simulink model "iBLF"  (R2015b)
settings: Solver=VariableStepAuto  StartTime=0.0  StopTime=10.0  RelTol=1e-3
settings Model: Creator=raghavv  LastModifiedBy=raghavv

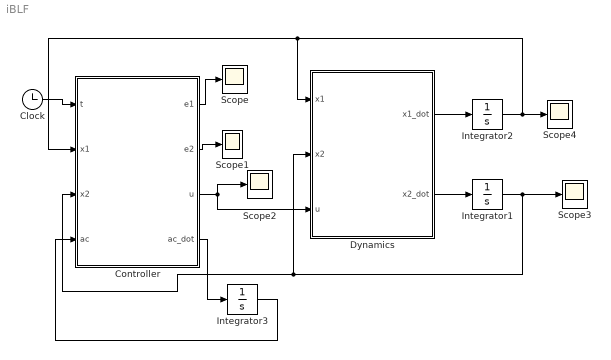
== system iBLF ==
  Clock : Clock
      settings: Decimation=50
  Controller : MATLAB Function  TreatAsAtomicUnit=on
  Dynamics : MATLAB Function  TreatAsAtomicUnit=on
  Integrator1 : Integrator  InitialCondition=2.0
  Integrator2 : Integrator  InitialCondition=0.5
  Integrator3 : Integrator
  Scope{,1..4} (5 alike) : Scope
  wires:
  Controller/3(u) -> Scope2/1, Dynamics/3(u)
  Controller/1(e1) -> Scope/1
  Controller/2(e2) -> Scope1/1
  Dynamics/1(x1_dot) -> Integrator2/1
  Dynamics/2(x2_dot) -> Integrator1/1
  Integrator2/1 -> Scope4/1, Dynamics/1(x1), Controller/2(x1)
  Integrator1/1 -> Scope3/1, Controller/3(x2), Dynamics/2(x2)
  Clock/1 -> Controller/1(t)
  Controller/4(ac_dot) -> Integrator3/1
  Integrator3/1 -> Controller/4(ac)

== matlab function iBLF/Controller ==
  data: t input; e1 output; e2 output; u output; x1 input; x2 input; ac input; ac_dot output
function [e1,e2,u,ac_dot] = Controller(t,x1,x2,ac)
%#codegen

theta1 = 0.1;
theta2 = 0.1;
theta3 = -0.2;

kc1 = 1.0;
kc2 = 2.5;

k1 = 5;
k2 = 5;

x1_dot = theta1*x1^2 + x2;
%x2_dot = theta2*x1*x2 + theta3*x1 + (1 + x1^2)*u;

yd = 0.2*sin(2.5*t);
yd_dot = 0.2*2.5*cos(2.5*t);
yd_ddot = -0.2*2.5^2*sin(2.5*t);

%WORKING
% yd = 0.2;
% yd_dot = 0;
% yd_ddot = 0;

z1 = x1-yd;
z1_dot = x1_dot-yd_dot;

%tau1 = (kc1/(2*z1))*log((kc1+z1+yd)*(kc1-yd)/((kc1-z1-yd)*(kc1+yd)));
if abs(z1) == 0
    tau1 = kc1^2/(kc1^2-yd^2);
    tau1_dot_dz = kc1/2*(1/(kc1+z1+yd)^2 + 1/(kc1-z1-yd)^2);
else    
    tau1 = (kc1/(2*z1))*log((kc1+z1+yd)*(kc1-yd)/((kc1-z1-yd)*(kc1+yd)));
    tau1_dot_dz = (1/z1)*(kc1^2/(kc1^2-(z1+yd)^2)-tau1)*z1_dot;
end


tau1_dot = tau1_dot_dz + yd_dot*kc1^2*(z1+2*yd)/(kc1^2-(z1+yd)^2)/(kc1^2-yd^2);

a1 = -theta1*(x1^2)-k1*z1+yd_dot*(kc1^2-x1^2)*tau1/(kc1^2);
z2 = x2 - a1;

%tau2 = (kc2/(2*z2))*log((kc2+z2+a1)*(kc2-a1)/((kc2-z2-a1)*(kc2+a1)));
if abs(z2) == 0
   tau2 = kc2^2/(kc2^2-a1^2);
else
    tau2 = (kc2/(2*z2))*log((kc2+z2+a1)*(kc2-a1)/((kc2-z2-a1)*(kc2+a1)));
end

%a1_dot is not used when Dynamic Surface Approximation done
a1_dot = -theta1*(2*x1*x1_dot)-k1*z1_dot + yd_dot*(kc1^2-x1^2)*tau1_dot/(kc1^2) - 2*yd_dot*x1*x1_dot*tau1/(kc1^2) + yd_ddot*(kc1^2-x1^2)*tau1/(kc1^2);
%comment ac_dot and replace ac with a1 for NO Dynamic Surface Approx.
gamma = 0.02;
ac_dot = 1/gamma*(-ac + a1);
u = 1/(1+x1^2)*(-theta3*x1-theta2*x1*x2-k2*z2+ac_dot*tau2*(kc2^2-x2^2)/kc2^2-(kc2^2-x2^2)*kc1^2*z1/(kc1^2-x1^2)/kc2^2);


e1 = x1 - yd;
e2 = x2 - yd_dot;

== matlab function iBLF/Dynamics ==
  data: x1 input; x1_dot output; x2 input; x2_dot output; u input
function [x1_dot,x2_dot] = Dynamics(x1,x2,u)
%#codegen

theta1 = 0.1;
theta2 = 0.1;
theta3 = -0.2;



x1_dot = theta1*x1^2 + x2;

x2_dot = theta2*x1*x2 + theta3*x1 + (1 + x1^2)*u;
